simulink model "ex2_sim"  (R2014b)
settings: Solver=ode45  StartTime=0.0  StopTime=2  RelTol=1e-3
undefined symbols (not defined in the file): d, freq, k, m
settings Model: Creator=gabras  LastModifiedBy=gabras

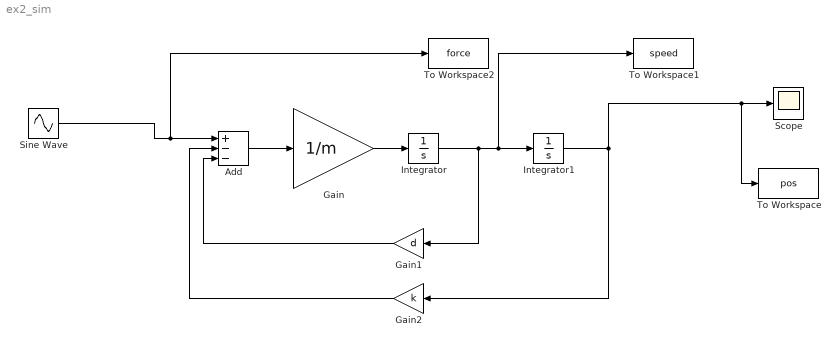
== system ex2_sim ==
  Add : Sum  Inputs=+--
  Gain : Gain  Gain=1/m
  Gain1 : Gain  Gain=d
  Gain2 : Gain  Gain=k
  Integrator : Integrator
  Integrator1 : Integrator
  Scope : Scope
  Sine Wave : Sin  Frequency=freq  SampleTime=0
  To Workspace : ToWorkspace  VariableName=pos  SaveFormat=Timeseries  SampleTime=-1
  To Workspace1 : ToWorkspace  VariableName=speed  SaveFormat=Timeseries  SampleTime=-1
  To Workspace2 : ToWorkspace  VariableName=force  SaveFormat=Timeseries  SampleTime=-1
  wires:
  Sine Wave/1 -> To Workspace2/1, Add/1
  Add/1 -> Gain/1
  Gain/1 -> Integrator/1
  Integrator/1 -> Gain1/1, To Workspace1/1, Integrator1/1
  Integrator1/1 -> To Workspace/1, Scope/1, Gain2/1
  Gain1/1 -> Add/3
  Gain2/1 -> Add/2
